simulink library "INT_EngTrqPtd_CoOfs"  (R2016b)
settings: Solver=VariableStepAuto  StartTime=0.0  StopTime=10.0  RelTol=1e-3
settings Model: Creator=Administrator  LastModifiedBy=Administrator

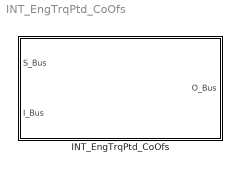
== system INT_EngTrqPtd_CoOfs ==
  INT_EngTrqPtd_CoOfs : Subsystem

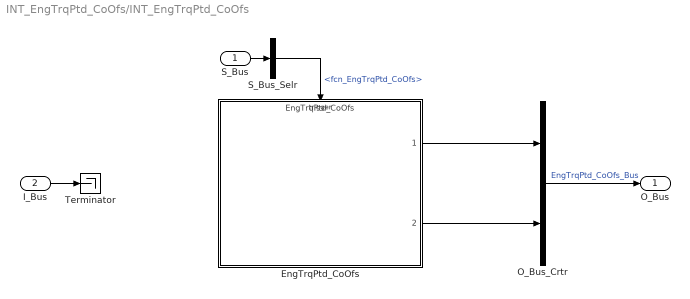
== system INT_EngTrqPtd_CoOfs/INT_EngTrqPtd_CoOfs ==
  S_Bus : Inport
  I_Bus : Inport  Port=2
  EngTrqPtd_CoOfs : ModelReference  ModelNameDialog=EngTrqPtd_CoOfs  SimulationMode=Normal  ModelReferenceVersion=1.2  TriggerPortName=function  TriggerPortTriggerType=function-call  TriggerPortStatesWhenEnabling=held
  O_Bus_Crtr : BusCreator  Inputs=2
  S_Bus_Selr : BusSelector  OutputSignals=fcn_EngTrqPtd_CoOfs
  Terminator : Terminator
  O_Bus : Outport
  wires:
  S_Bus_Selr/1 -> EngTrqPtd_CoOfs/Trigger  "<fcn_EngTrqPtd_CoOfs>"
  S_Bus/1 -> S_Bus_Selr/1
  I_Bus/1 -> Terminator/1
  O_Bus_Crtr/1 -> O_Bus/1  "EngTrqPtd_CoOfs_Bus"
  EngTrqPtd_CoOfs/1 -> O_Bus_Crtr/1
  EngTrqPtd_CoOfs/2 -> O_Bus_Crtr/2
